simulink model "sampleModel1437"  (R2023a)
settings: Solver=VariableStepAuto  StartTime=0.0  StopTime=10.0  RelTol=1e-3
libraries: hdlsllib x6
settings Model: Creator=user1  LastModifiedBy=user1

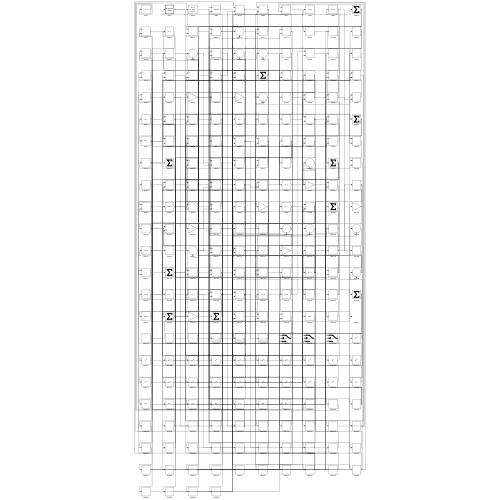
[thumbnail: Simulink's stored preview of the top-level diagram]
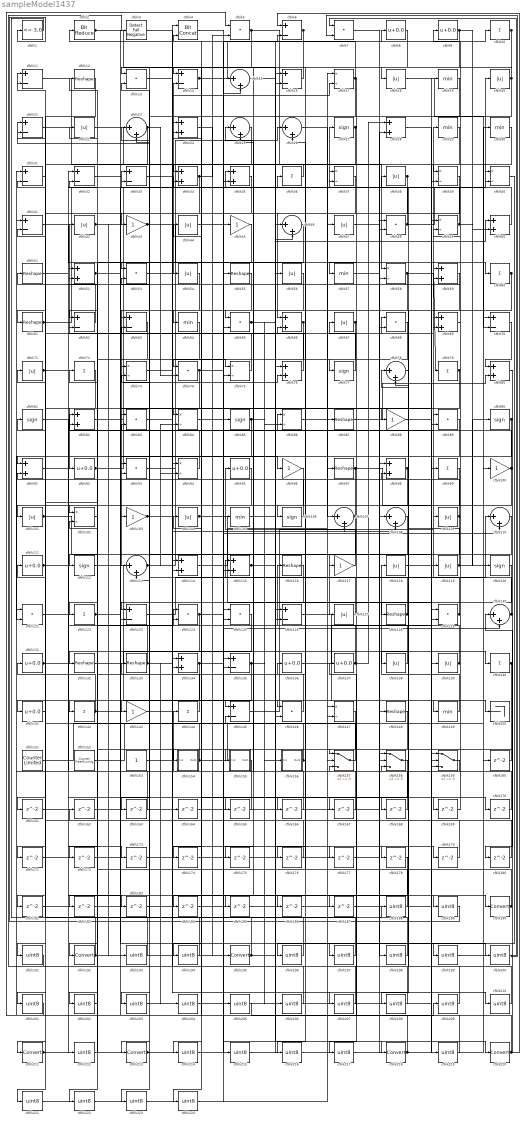
== system sampleModel1437 ==
  cfblk1 : hdlsllib/Logic and Bit Operations/Compare To Constant  relop=<=  const=3.0  OutDataTypeStr=boolean
  cfblk{10,36,60,72,79,99,122,140,142,144} (10 alike) : Sum  Inputs=+
  cfblk{43,45,88,96,100,103,117,143} (8 alike) : Gain
  cfblk{18,20,22,38,42,44,47,54,56,67,71,101,104,109,118..119,127,138..139} (19 alike) : Abs  SaturateOnIntegerOverflow=off
  cfblk{17,37,39..40,49,58,73,75,84,86,94,102,147} (13 alike) : Product  Inputs=*/  RndMeth=Zero  SaturateOnIntegerOverflow=on
  cfblk{19,29..30,57,64,105,149} (7 alike) : MinMax
  cfblk{27,77,81,85,90,106,112,120} (8 alike) : Signum
  cfblk{15,23,25..26,46,78,107..108,110,113,130} (11 alike) : Sum  Inputs=|++
  cfblk{6,11,14,16,21,31..33,41,62..63,70,123,126,135,145} (16 alike) : Sum  Inputs=+-
  cfblk{8..9,92,95,111,131,136..137,141} (9 alike) : Bias  Bias=0.0  SaturateOnIntegerOverflow=off
  cfblk{24,28,34..35,50,52,59,66,69,76,80,82,91,98,114..115,134} (17 alike) : Sum
  cfblk{12,51,55,61,87,97,116,128,132..133,148} (11 alike) : Reshape
  cfblk{5,7,13,48,53,65,68,74,83,89,93,121,124..125,129,146} (16 alike) : DotProduct  OutDataTypeStr=Inherit: Inherit via internal rule
  cfblk150 : Terminator
  cfblk151 : hdlsllib/Sources/Counter Limited  uplimit=7  tsamp=-1
  cfblk152 : hdlsllib/Sources/Counter Free-Running  NumBits=16  tsamp=-1
  cfblk153 : Constant  SampleTime=-1
  cfblk154 : Subsystem
      settings: LibrarySourceBlock=|
      | hdlsllib/Ports &
      | Subsystems/Subsystem
  cfblk155 : Subsystem
      settings: LibrarySourceBlock=|
      | hdlsllib/Ports &
      | Subsystems/Subsystem
  cfblk156 : Subsystem
      settings: LibrarySourceBlock=|
      | hdlsllib/Ports &
      | Subsystems/Subsystem
  cfblk157 : Switch  SaturateOnIntegerOverflow=off  InputSameDT=off
  cfblk158 : Switch  SaturateOnIntegerOverflow=off  InputSameDT=off
  cfblk159 : Switch  SaturateOnIntegerOverflow=off  InputSameDT=off
  cfblk{160..187} (28 alike) : Delay  SampleTime=1
  cfblk{188..189,191,193..194,196..210,212,214..217,219,221..224} (30 alike) : DataTypeConversion  OutDataTypeStr=uint8  SaturateOnIntegerOverflow=off  RndMeth=Floor
  cfblk{190,192,195,211,213,218,220} (7 alike) : DataTypeConversion  SaturateOnIntegerOverflow=off  RndMeth=Floor
  cfblk2 : hdlsllib/Logic and Bit Operations/Bit Reduce  mode=AND
  cfblk3 : hdlsllib/Logic and Bit Operations/Detect Fall Negative  vinit=0  OutDataTypeStr=boolean
  cfblk4 : hdlsllib/Logic and Bit Operations/Bit Concat  numInputs=2
  wires:
  cfblk134/1 -> cfblk110/2, cfblk171/1, cfblk177/1
  cfblk49/1 -> cfblk33/1, cfblk50/2
  cfblk107/1 -> cfblk102/1, cfblk126/2
  cfblk50/1 -> cfblk14/1
  cfblk129/1 -> cfblk29/1, cfblk21/2
  cfblk9/1 -> cfblk120/1, cfblk174/1
  cfblk14/1 -> cfblk8/1, cfblk130/2
  cfblk61/1 -> cfblk36/1, cfblk34/2
  cfblk29/1 -> cfblk39/1
  cfblk24/1 -> cfblk195/1
  cfblk77/1 -> cfblk67/1
  cfblk70/1 -> cfblk80/1
  cfblk147/1 -> cfblk213/1
  cfblk52/1 -> cfblk141/1, cfblk96/1
  cfblk26/1 -> cfblk87/1
  cfblk117/1 -> cfblk95/1
  cfblk47/1 -> cfblk148/1
  cfblk155/1(Out1) -> cfblk144/1
  cfblk92/1 -> cfblk14/2, cfblk55/1
  cfblk5/1 -> cfblk107/1, cfblk35/2
  cfblk62/1 -> cfblk51/1
  cfblk143/1 -> cfblk149/1
  cfblk75/1 -> cfblk42/1
  cfblk87/1 -> cfblk80/2
  cfblk122/1 -> cfblk166/1, cfblk167/1
  cfblk113/1 -> cfblk26/1, cfblk94/2
  cfblk104/1 -> cfblk159/1, cfblk6/2
  cfblk41/1 -> cfblk60/1
  cfblk31/1 -> cfblk61/1
  cfblk144/1 -> cfblk52/1
  cfblk152/1 -> cfblk105/1
  cfblk11/1 -> cfblk58/1
  cfblk18/1 -> cfblk70/1
  cfblk34/1 -> cfblk101/1, cfblk5/2
  cfblk149/1 -> cfblk118/1
  cfblk51/1 -> cfblk38/1
  cfblk28/1 -> cfblk139/1
  cfblk48/1 -> cfblk20/1, cfblk37/2
  cfblk114/1 -> cfblk97/1
  cfblk36/1 -> cfblk34/1
  cfblk65/1 -> cfblk69/2, cfblk206/1
  cfblk151/1 -> cfblk16/1
  cfblk142/1 -> cfblk81/1, cfblk37/1, cfblk124/1
  cfblk106/1 -> cfblk11/1
  cfblk133/1 -> cfblk102/2, cfblk204/1, cfblk210/1
  cfblk112/1 -> cfblk145/1
  cfblk93/1 -> cfblk27/1
  cfblk72/1 -> cfblk211/1
  cfblk66/1 -> cfblk125/2, cfblk165/1
  cfblk17/1 -> cfblk2/1, cfblk57/1, cfblk154/1(In1)
  cfblk59/1 -> cfblk64/1
  cfblk74/1 -> cfblk92/1, cfblk146/1
  cfblk20/1 -> cfblk43/1, cfblk18/1, cfblk185/1
  cfblk126/1 -> cfblk150/1
  cfblk132/1 -> cfblk140/1
  cfblk145/1 -> cfblk109/1
  cfblk103/1 -> cfblk84/2, cfblk178/1
  cfblk109/1 -> cfblk138/1, cfblk25/2
  cfblk60/1 -> cfblk88/1, cfblk217/1
  cfblk37/1 -> cfblk74/1
  cfblk56/1 -> cfblk113/1
  cfblk33/1 -> cfblk54/1
  cfblk89/1 -> cfblk112/1
  cfblk38/1 -> cfblk66/1, cfblk197/1
  cfblk27/1 -> cfblk73/1, cfblk84/1
  cfblk105/1 -> cfblk56/1
  cfblk83/1 -> cfblk114/1
  cfblk137/1 -> cfblk32/2, cfblk13/2, cfblk28/1
  cfblk13/1 -> cfblk108/2
  cfblk10/1 -> cfblk65/1, cfblk176/1
  cfblk22/1 -> cfblk46/1
  cfblk130/1 -> cfblk66/2, cfblk86/1
  cfblk2/1 -> cfblk16/2, cfblk89/2
  cfblk128/1 -> cfblk73/2, cfblk62/2, cfblk98/2
  cfblk157/1 -> cfblk82/1
  cfblk102/1 -> cfblk122/1
  cfblk96/1 -> cfblk106/1
  cfblk82/1 -> cfblk76/2
  cfblk6/1 -> cfblk143/1, cfblk115/2
  cfblk8/1 -> cfblk53/1
  cfblk135/1 -> cfblk156/1(In1), cfblk191/1
  cfblk123/1 -> cfblk110/1
  cfblk154/1(Out1) -> cfblk21/1, cfblk30/1
  cfblk85/1 -> cfblk121/2, cfblk86/2
  cfblk140/1 -> cfblk186/1, cfblk187/1
  cfblk97/1 -> cfblk129/1, cfblk161/1
  cfblk30/1 -> cfblk77/1
  cfblk118/1 -> cfblk40/1
  cfblk53/1 -> cfblk75/1
  cfblk55/1 -> cfblk65/2
  cfblk101/1 -> cfblk135/1, cfblk71/1, cfblk129/2
  cfblk69/1 -> cfblk9/1
  cfblk138/1 -> cfblk53/2
  cfblk3/1 -> cfblk190/1
  cfblk76/1 -> cfblk41/2
  cfblk139/1 -> cfblk116/1, cfblk59/2
  cfblk110/1 -> cfblk127/1
  cfblk43/1 -> cfblk70/2, cfblk17/2
  cfblk25/1 -> cfblk75/2
  cfblk98/1 -> cfblk103/1, cfblk194/1
  cfblk79/1 -> cfblk123/2, cfblk181/1, cfblk182/1
  cfblk86/1 -> cfblk68/1
  cfblk64/1 -> cfblk132/1
  cfblk44/1 -> cfblk218/1
  cfblk108/1 -> cfblk113/2
  cfblk100/1 -> cfblk52/2, cfblk142/1
  cfblk67/1 -> cfblk155/1(In1), cfblk184/1
  cfblk141/1 -> cfblk11/2
  cfblk16/1 -> cfblk13/1
  cfblk71/1 -> cfblk59/1, cfblk69/1
  cfblk127/1 -> cfblk115/1
  cfblk90/1 -> cfblk128/1, cfblk180/1
  cfblk23/1 -> cfblk91/1, cfblk74/2
  cfblk46/1 -> cfblk62/1
  cfblk124/1 -> cfblk107/2, cfblk134/2
  cfblk159/1 -> cfblk158/3
  cfblk136/1 -> cfblk49/1
  cfblk15/1 -> cfblk220/1
  cfblk94/1 -> cfblk23/1
  cfblk119/1 -> cfblk35/1, cfblk90/1
  cfblk116/1 -> cfblk123/1
  cfblk39/1 -> cfblk117/1
  cfblk54/1 -> cfblk83/1
  cfblk111/1 -> cfblk168/1, cfblk169/1
  cfblk146/1 -> cfblk133/1
  cfblk42/1 -> cfblk170/1, cfblk193/1
  cfblk21/1 -> cfblk46/2
  cfblk115/1 -> cfblk50/1, cfblk10/1
  cfblk131/1 -> cfblk89/1, cfblk124/2
  cfblk58/1 -> cfblk79/1, cfblk68/2, cfblk93/2
  cfblk57/1 -> cfblk40/2
  cfblk63/1 -> cfblk192/1
  cfblk156/1(Out1) -> cfblk25/1, cfblk26/2
  cfblk160/1 -> cfblk157/1
  cfblk161/1 -> cfblk114/2
  cfblk80/1 -> cfblk162/1
  cfblk35/1 -> cfblk163/1
  cfblk163/1 -> cfblk82/2
  cfblk73/1 -> cfblk164/1
  cfblk164/1 -> cfblk108/1
  cfblk165/1 -> cfblk41/1
  cfblk166/1 -> cfblk32/1
  cfblk167/1 -> cfblk94/1
  cfblk168/1 -> cfblk145/2
  cfblk169/1 -> cfblk49/2
  cfblk170/1 -> cfblk31/2
  cfblk171/1 -> cfblk158/1
  cfblk148/1 -> cfblk172/1
  cfblk172/1 -> cfblk48/2
  cfblk121/1 -> cfblk173/1
  cfblk174/1 -> cfblk76/1
  cfblk120/1 -> cfblk175/1
  cfblk175/1 -> cfblk158/2
  cfblk176/1 -> cfblk91/2
  cfblk177/1 -> cfblk157/3
  cfblk84/1 -> cfblk179/1
  cfblk179/1 -> cfblk33/2
  cfblk180/1 -> cfblk23/2
  cfblk181/1 -> cfblk58/2
  cfblk182/1 -> cfblk135/2
  cfblk81/1 -> cfblk183/1
  cfblk183/1 -> cfblk17/1
  cfblk185/1 -> cfblk39/2
  cfblk186/1 -> cfblk159/2
  cfblk187/1 -> cfblk159/3
  cfblk1/1 -> cfblk188/1
  cfblk188/1 -> cfblk104/1
  cfblk153/1 -> cfblk189/1
  cfblk189/1 -> cfblk1/1
  cfblk190/1 -> cfblk22/1, cfblk83/2, cfblk136/1
  cfblk191/1 -> cfblk3/1
  cfblk192/1 -> cfblk126/1, cfblk111/1
  cfblk193/1 -> cfblk63/1
  cfblk194/1 -> cfblk63/2
  cfblk195/1 -> cfblk134/1, cfblk131/1
  cfblk40/1 -> cfblk196/1
  cfblk196/1 -> cfblk24/1
  cfblk197/1 -> cfblk24/2
  cfblk7/1 -> cfblk198/1
  cfblk198/1 -> cfblk48/1
  cfblk32/1 -> cfblk199/1
  cfblk199/1 -> cfblk7/1
  cfblk162/1 -> cfblk200/1
  cfblk200/1 -> cfblk7/2
  cfblk12/1 -> cfblk201/1
  cfblk201/1 -> cfblk5/1
  cfblk125/1 -> cfblk202/1
  cfblk202/1 -> cfblk12/1
  cfblk19/1 -> cfblk203/1
  cfblk203/1 -> cfblk125/1
  cfblk204/1 -> cfblk19/1
  cfblk4/1 -> cfblk205/1
  cfblk206/1 -> cfblk4/1
  cfblk173/1 -> cfblk207/1
  cfblk207/1 -> cfblk4/2
  cfblk78/1 -> cfblk208/1
  cfblk208/1 -> cfblk121/1
  cfblk205/1 -> cfblk209/1
  cfblk209/1 -> cfblk78/1
  cfblk210/1 -> cfblk78/2
  cfblk211/1 -> cfblk85/1, cfblk100/1, cfblk119/1
  cfblk91/1 -> cfblk212/1
  cfblk212/1 -> cfblk72/1
  cfblk213/1 -> cfblk28/2, cfblk146/2, cfblk157/2
  cfblk158/1 -> cfblk214/1
  cfblk214/1 -> cfblk147/1
  cfblk184/1 -> cfblk215/1
  cfblk215/1 -> cfblk147/2
  cfblk99/1 -> cfblk216/1
  cfblk216/1 -> cfblk160/1
  cfblk217/1 -> cfblk99/1
  cfblk218/1 -> cfblk98/1, cfblk93/1, cfblk31/1
  cfblk88/1 -> cfblk219/1
  cfblk219/1 -> cfblk44/1
  cfblk220/1 -> cfblk6/1, cfblk130/1, cfblk137/1
  cfblk95/1 -> cfblk221/1
  cfblk221/1 -> cfblk15/1
  cfblk178/1 -> cfblk222/1
  cfblk222/1 -> cfblk15/2
  cfblk45/1 -> cfblk223/1
  cfblk223/1 -> cfblk47/1
  cfblk68/1 -> cfblk224/1
  cfblk224/1 -> cfblk45/1

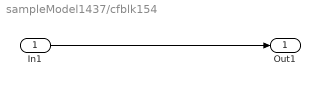
== system sampleModel1437/cfblk154 ==
  In1 : Inport
  Out1 : Outport
  wires:
  In1/1 -> Out1/1

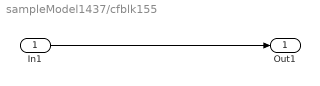
== system sampleModel1437/cfblk155 ==
  In1 : Inport
  Out1 : Outport
  wires:
  In1/1 -> Out1/1

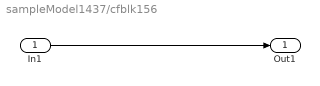
== system sampleModel1437/cfblk156 ==
  In1 : Inport
  Out1 : Outport
  wires:
  In1/1 -> Out1/1
